simulink model "lab_model"  (Simulink 7.6)
settings: Solver=ode45  StartTime=0.0  StopTime=10.0  RelTol=1e-3
undefined symbols (not defined in the file): J, Kcur_fdb, kcur_i, kcur_p, Ke, Km, Kpwc, Kspd_fdb, Kspd_p, R, Te, Tpwc
settings Model: Creator=Student  LastModifiedBy=pps  CovModelRefEnable=off
settings DataIOCC: LimitDataPoints=off  SaveFormat=StructureWithTime
settings OptimizationCC: ExpressionDepthLimit=128
settings DebuggingCC: UnderspecifiedInitializationDetection=Simplified  MergeDetectMultiDrivingBlocksExec=error  SolverPrmCheckMsg=none  FcnCallInpInsideContextMsg=Enable All  StateNameClashWarn=none
settings HardwareCC: ProdIntDivRoundTo=Zero  ProdEndianess=LittleEndian  ProdHWDeviceType=Specified
settings CodeAppCC: CustomSymbolStrType=$N$R$M_T
settings GRTTargetCC: TargetFunctionLibrary=C89/C90 (ANSI)

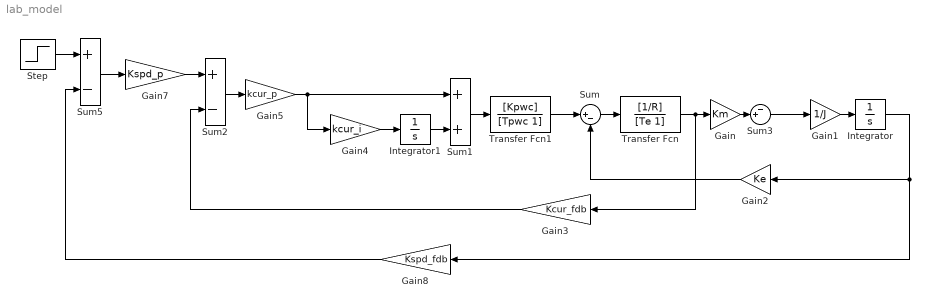
== system lab_model ==
  Gain : Gain  Gain=Km
  Gain1 : Gain  Gain=1/J
  Gain2 : Gain  Gain=Ke
  Gain3 : Gain  Gain=Kcur_fdb
  Gain4 : Gain  Gain=kcur_i
  Gain5 : Gain  Gain=kcur_p
  Gain7 : Gain  Gain=Kspd_p
  Gain8 : Gain  Gain=Kspd_fdb
  Integrator : Integrator
  Integrator1 : Integrator
  Step : Step  Time=0  SampleTime=0
  Sum : Sum  Inputs=|+-
  Sum1 : Sum
  Sum2 : Sum  Inputs=+-
  Sum3 : Sum  Inputs=-+|
  Sum5 : Sum  Inputs=+-
  Transfer Fcn : TransferFcn  Numerator=[1/R]  Denominator=[Te 1]
  Transfer Fcn1 : TransferFcn  Numerator=[Kpwc]  Denominator=[Tpwc 1]
  wires:
  Transfer Fcn/1 -> Gain3/1, Gain/1
  Gain1/1 -> Integrator/1
  Sum/1 -> Transfer Fcn/1
  Gain2/1 -> Sum/2
  Integrator/1 -> Gain8/1, Gain2/1
  Transfer Fcn1/1 -> Sum/1
  Sum1/1 -> Transfer Fcn1/1
  Integrator1/1 -> Sum1/2
  Gain4/1 -> Integrator1/1
  Gain5/1 -> Gain4/1, Sum1/1
  Sum2/1 -> Gain5/1
  Gain3/1 -> Sum2/2
  Gain/1 -> Sum3/2
  Sum3/1 -> Gain1/1
  Sum5/1 -> Gain7/1
  Gain8/1 -> Sum5/2
  Gain7/1 -> Sum2/1
  Step/1 -> Sum5/1
